simulink model "MuxVsBus"  (R2025b)
settings: Solver=FixedStepDiscrete  StartTime=0.0  StopTime=10.0  FixedStep=0.01  RelTol=1e-3
settings Model: Creator=soura  LastModifiedBy=soura
settings OptimizationCC: DefaultParameterBehavior=Inlined  EnhancedBackFolding=on  PassReuseOutputArgsAs=Individual arguments  ZeroExternalMemoryAtStartup=off  ZeroInternalMemoryAtStartup=off  OptimizeBlockOrder=speed  DifferentSizesBufferReuse=on  OptimizationCustomize=off  EfficientTunableParamExpr=on
settings DebuggingCC: ParameterTunabilityLossMsg=error
settings SFSimCC: MATLABDynamicMemAlloc=off
settings RTWCC: SystemTargetFile=ert.tlc  GenCodeOnly=on  TemplateMakefile=ert_default_tmf  Description=Embedded Coder
settings CodeAppCC: ForceParamTrailComments=on  IgnoreCustomStorageClasses=off  OperatorAnnotations=on  SimulinkDataObjDesc=on  SFDataObjDesc=on  InsertBlockDesc=on
settings ERTTargetCC: ERTCustomFileTemplate=example_file_process.tlc  ERTFilePackagingFormat=CompactWithDataFile  TargetLangStandard=C99 (ISO)  GenerateSampleERTMain=on

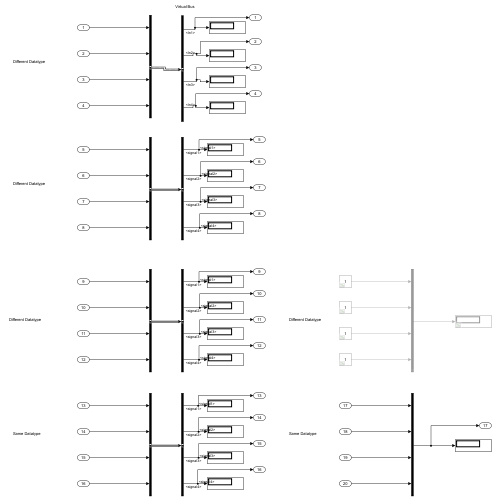
[thumbnail: Simulink's stored preview of the top-level diagram]
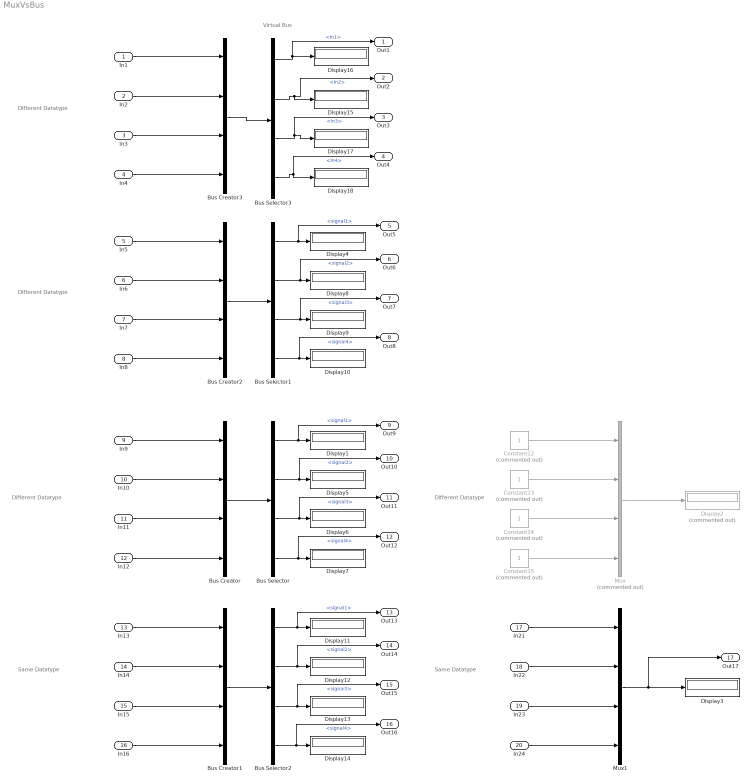
== system MuxVsBus ==
  note: Virtual Bus
  note: Different Datatype
  note: Different Datatype
  note: Different Datatype
  note: Same Datatype
  note: Same Datatype
  note: Different Datatype
  In1 : Inport  OutDataTypeStr=boolean
  In2 : Inport  Port=2  OutDataTypeStr=uint8
  In3 : Inport  Port=3  OutDataTypeStr=int16
  In4 : Inport  Port=4  OutDataTypeStr=single
  In5 : Inport  Port=5  OutDataTypeStr=boolean
  In6 : Inport  Port=6  OutDataTypeStr=uint8
  In7 : Inport  Port=7  OutDataTypeStr=int16
  In8 : Inport  Port=8  OutDataTypeStr=single
  In9 : Inport  Port=9  OutDataTypeStr=boolean
  In10 : Inport  Port=10  OutDataTypeStr=uint8
  In11 : Inport  Port=11  OutDataTypeStr=int16
  In12 : Inport  Port=12  OutDataTypeStr=single
  In13 : Inport  Port=13  OutDataTypeStr=boolean
  In14 : Inport  Port=14  OutDataTypeStr=boolean
  In15 : Inport  Port=15  OutDataTypeStr=boolean
  In16 : Inport  Port=16  OutDataTypeStr=boolean
  In21 : Inport  Port=17  OutDataTypeStr=boolean
  In22 : Inport  Port=18  OutDataTypeStr=boolean
  In23 : Inport  Port=19  OutDataTypeStr=boolean
  In24 : Inport  Port=20  OutDataTypeStr=boolean
  Bus Creator : BusCreator  Inputs=4
  Bus Creator1 : BusCreator  Inputs=4
  Bus Creator2 : BusCreator  Inputs=4
  Bus Creator3 : BusCreator  Inputs=4  OutDataTypeStr=Bus: BS  NonVirtualBus=on
      settings: InheritFromInputs=off
  Bus Selector : BusSelector  OutputSignals=signal1,signal2,signal3,signal4
  Bus Selector1 : BusSelector  OutputSignals=signal1,signal2,signal3,signal4
  Bus Selector2 : BusSelector  OutputSignals=signal1,signal2,signal3,signal4
  Bus Selector3 : BusSelector  OutputSignals=In1,In2,In3,In4
  Constant12 : Constant  Commented=on  OutDataTypeStr=boolean
  Constant13 : Constant  Commented=on  OutDataTypeStr=uint8
  Constant14 : Constant  Commented=on  OutDataTypeStr=int16
  Constant15 : Constant  Commented=on  OutDataTypeStr=single
  Display{1,3..18} (17 alike) : Display
  Display2 : Display  Commented=on
  Mux : Mux  Commented=on
  Mux1 : Mux
  Out1 : Outport
  Out2 : Outport  Port=2
  Out3 : Outport  Port=3
  Out4 : Outport  Port=4
  Out5 : Outport  Port=5
  Out6 : Outport  Port=6
  Out7 : Outport  Port=7
  Out8 : Outport  Port=8
  Out9 : Outport  Port=9
  Out10 : Outport  Port=10
  Out11 : Outport  Port=11
  Out12 : Outport  Port=12
  Out13 : Outport  Port=13
  Out14 : Outport  Port=14
  Out15 : Outport  Port=15
  Out16 : Outport  Port=16
  Out17 : Outport  Port=17
  wires:
  In9/1 -> Bus Creator/1
  In10/1 -> Bus Creator/2
  In11/1 -> Bus Creator/3
  In12/1 -> Bus Creator/4
  In16/1 -> Bus Creator1/4
  In15/1 -> Bus Creator1/3
  In14/1 -> Bus Creator1/2
  In13/1 -> Bus Creator1/1
  In8/1 -> Bus Creator2/4
  In7/1 -> Bus Creator2/3
  In6/1 -> Bus Creator2/2
  In5/1 -> Bus Creator2/1
  In21/1 -> Mux1/1
  In22/1 -> Mux1/2
  In23/1 -> Mux1/3
  In24/1 -> Mux1/4
  Constant15/1 -> Mux/4
  Constant14/1 -> Mux/3
  Constant13/1 -> Mux/2
  Constant12/1 -> Mux/1
  Mux/1 -> Display2/1
  Mux1/1 -> Out17/1, Display3/1
  Bus Creator/1 -> Bus Selector/1
  Bus Creator2/1 -> Bus Selector1/1
  Bus Creator1/1 -> Bus Selector2/1
  Bus Creator3/1 -> Bus Selector3/1
  Bus Selector3/1 -> Out1/1, Display16/1  "<In1>"
  In1/1 -> Bus Creator3/1
  In2/1 -> Bus Creator3/2
  In3/1 -> Bus Creator3/3
  In4/1 -> Bus Creator3/4
  Bus Selector3/4 -> Out4/1, Display18/1  "<In4>"
  Bus Selector3/3 -> Out3/1, Display17/1  "<In3>"
  Bus Selector3/2 -> Out2/1, Display15/1  "<In2>"
  Bus Selector1/2 -> Out6/1, Display8/1  "<signal2>"
  Bus Selector1/3 -> Out7/1, Display9/1  "<signal3>"
  Bus Selector1/4 -> Out8/1, Display10/1  "<signal4>"
  Bus Selector1/1 -> Out5/1, Display4/1  "<signal1>"
  Bus Selector/1 -> Out9/1, Display1/1  "<signal1>"
  Bus Selector/4 -> Out12/1, Display7/1  "<signal4>"
  Bus Selector/3 -> Out11/1, Display6/1  "<signal3>"
  Bus Selector/2 -> Out10/1, Display5/1  "<signal2>"
  Bus Selector2/2 -> Out14/1, Display12/1  "<signal2>"
  Bus Selector2/3 -> Out15/1, Display13/1  "<signal3>"
  Bus Selector2/4 -> Out16/1, Display14/1  "<signal4>"
  Bus Selector2/1 -> Out13/1, Display11/1  "<signal1>"
